simulink model "PID_control"  (R2021a)
settings: Solver=VariableStepAuto  StartTime=0.0  StopTime=50  RelTol=1e-3
libraries: pid_lib x1
settings Model: Creator=hty  LastModifiedBy=hty

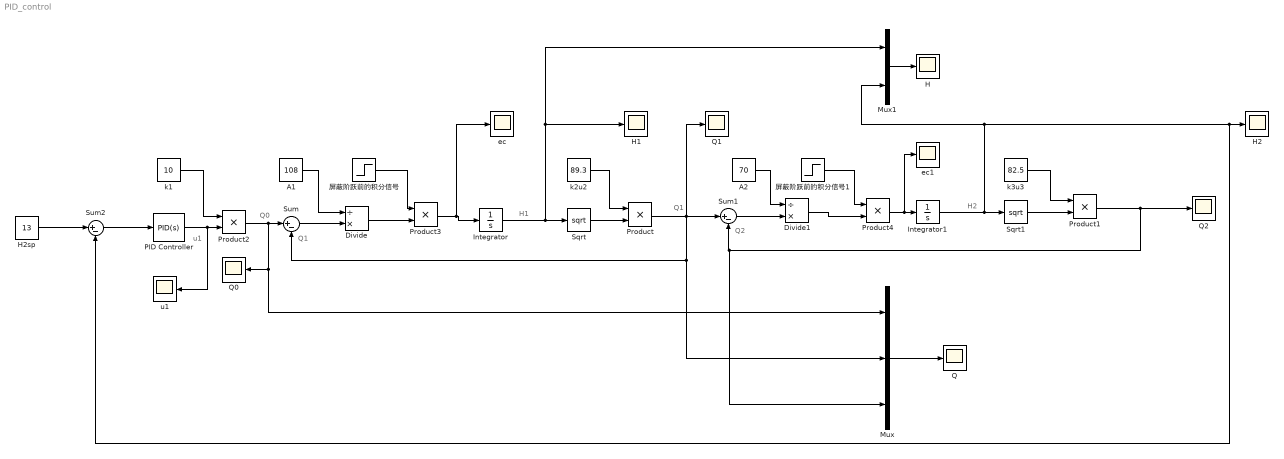
== system PID_control ==
  note: u1
  note: Q1
  note: Q1
  note: Q0
  note: H1
  note: Q2
  note: H2
  A1 : Constant  Value=108
  A2 : Constant  Value=70
  Divide : Product  Inputs=/*
  Divide1 : Product  Inputs=/*
  H : Scope
  H1 : Scope
  H2 : Scope
  H2sp : Constant  Value=13
  Integrator : Integrator  InitialCondition=10
  Integrator1 : Integrator  InitialCondition=13
  Mux : Mux  Inputs=3
  Mux1 : Mux  Inputs=2
  PID Controller : pid_lib/PID Controller  Controller=PID  Form=Parallel  TimeDomain=Continuous-time  UseExternalTs=off  SampleTime=-1  IntegratorMethod=Forward Euler  FilterMethod=Forward Euler  ControllerParametersSource=internal  P=100  I=1.  D=10  UseFilter=on  N=100  TunerSelectOption=Transfer Function Based (PID Tuner App)  InitialConditionSource=internal  InitialConditionForIntegrator=29.75  InitialConditionForFilter=0  DifferentiatorICPrevScaledInput=0  ExternalReset=none  TrackingMode=off  Kt=1  LimitOutput=off  SatLimitsSource=internal  UpperSaturationLimit=inf  LowerSaturationLimit=-inf  LinearizeAsGain=on  AntiWindupMode=none  Kb=1  POutMin=[]  POutMax=[]  IOutMin=[]  IOutMax=[]  DOutMin=[]  DOutMax=[]  NOutMin=[]  NOutMax=[]  SumOutMin=[]  SumOutMax=[]  SaturationOutMin=[]  SaturationOutMax=[]  PParamMin=[]  PParamMax=[]  IParamMin=[]  IParamMax=[]  DParamMin=[]  DParamMax=[]  NParamMin=[]  NParamMax=[]  KbParamMin=[]  KbParamMax=[]  KtParamMin=[]  KtParamMax=[]  KbOutMin=[]  KbOutMax=[]  KtOutMin=[]  KtOutMax=[]  IntegratorOutMin=[]  IntegratorOutMax=[]  FilterOutMin=[]  FilterOutMax=[]  SumI1OutMin=[]  SumI1OutMax=[]  SumI2OutMin=[]  SumI2OutMax=[]  SumI3OutMin=[]  SumI3OutMax=[]  SumI4OutMin=[]  SumI4OutMax=[]  SumDOutMin=[]  SumDOutMax=[]  DifferentiatorOutMin=[]  DifferentiatorOutMax=[]  FilterDiffOutCoefMin=[]  FilterDiffOutCoefMax=[]  ReciprocalOutMin=[]  ReciprocalOutMax=[]  SumDenOutMin=[]  SumDenOutMax=[]  SumNumOutMin=[]  SumNumOutMax=[]  DivideOutMin=[]  DivideOutMax=[]  UdiffTsProdOutMin=[]  UdiffTsProdOutMax=[]  NTsProdOutMin=[]  NTsProdOutMax=[]  UintegralTsProdOutMin=[]  UintegralTsProdOutMax=[]  UngainTsProdOutMin=[]  UngainTsProdOutMax=[]  IntegratorContinuousStateAttributes=''  IntegratorStateMustResolveToSignalObject=off  IntegratorRTWStateStorageClass=Auto  FilterContinuousStateAttributes=''  FilterStateMustResolveToSignalObject=off  FilterRTWStateStorageClass=Auto  ParallelPVariant=InternalParameters  IdealPVariant=Disabled  IVariant=InternalParameters  DVariant=InternalParameters  IntegratorVariant=Continuous  SatVariant=Disabled  AWVariant=Passthrough  PCopyVariant=Disabled  TRVariant=Disabled  FdbkBlocksVariant=Forward  IdealPFdbkVariant=Disabled  SatFdbkVariant=Disabled  DerivativeFilterVariant=ContFilter  NVariant=InternalParameters  NCopyVariant=Disabled  FilterICVariant=InternalICsFilter  IntegratorICVariant=InternalICs  ExternalResetVariant=Disabled  TRSumVariant=Passthrough  SumFdbkVariant=Disabled  SumVariant=Sum_PID  TsampFilterVariant=InternalTs  TsampNgainVariant=Passthrough  TsampIntegralVariant=Passthrough  ExternalSaturationOutDataTypeStr=Inherit: Same as second input
  Product{,1..4} (5 alike) : Product
  Q{,0..2} (4 alike) : Scope
  Sqrt : Sqrt  SaturateOnIntegerOverflow=on
  Sqrt1 : Sqrt  SaturateOnIntegerOverflow=on
  Sum : Sum  Inputs=|+-
  Sum1 : Sum  Inputs=|+-
  Sum2 : Sum  Inputs=|+-
  ec : Scope
  ec1 : Scope
  k1 : Constant  Value=10
  k2u2 : Constant  Value=89.3
  k3u3 : Constant  Value=82.5
  u1 : Scope
  屏蔽阶跃前的积分信号 : Step  Time=5  SampleTime=0
  屏蔽阶跃前的积分信号1 : Step  Time=5  SampleTime=0
  wires:
  Mux/1 -> Q/1
  Product4/1 -> ec1/1, Integrator1/1
  k1/1 -> Product2/1
  Sum1/1 -> Divide1/2
  Mux1/1 -> H/1
  k2u2/1 -> Product/1
  k3u3/1 -> Product1/1
  屏蔽阶跃前的积分信号/1 -> Product3/1
  Divide1/1 -> Product4/2
  A1/1 -> Divide/1
  Integrator1/1 -> Sum2/2, H2/1, Mux1/2, Sqrt1/1
  Product/1 -> Mux/2, Sum/2, Q1/1, Sum1/1
  屏蔽阶跃前的积分信号1/1 -> Product4/1
  A2/1 -> Divide1/1
  PID Controller/1 -> u1/1, Product2/2
  Product3/1 -> ec/1, Integrator/1
  Sqrt1/1 -> Product1/2
  Integrator/1 -> Mux1/1, H1/1, Sqrt/1
  Divide/1 -> Product3/2
  Sum/1 -> Divide/2
  Product2/1 -> Mux/1, Q0/1, Sum/1
  Sqrt/1 -> Product/2
  Product1/1 -> Mux/3, Sum1/2, Q2/1
  Sum2/1 -> PID Controller/1
  H2sp/1 -> Sum2/1
